simulink model "Problema4"  (R2023b)
settings: Solver=ode45  StartTime=0  StopTime=50  FixedStep=1  RelTol=1e-3
values from neighbouring files (symbols this model uses):
  constants = {    [sim_utils.m]
settings Model: Creator=alfre  LastModifiedBy=alfre

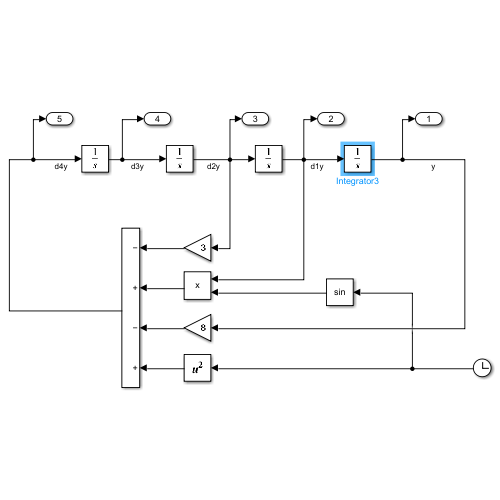
[thumbnail: Simulink's stored preview of the top-level diagram]
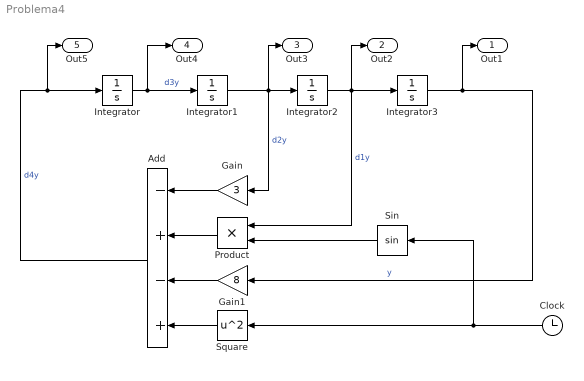
== system Problema4 ==
  Add : Sum  Inputs=-+-+
  Clock : Clock
  Gain : Gain  Gain=3
  Gain1 : Gain  Gain=8
  Integrator : Integrator  InitialCondition=constants{1}.d3y0
  Integrator1 : Integrator  InitialCondition=constants{1}.d2y0
  Integrator2 : Integrator  InitialCondition=constants{1}.dy0
  Integrator3 : Integrator  InitialCondition=constants{1}.y0
  Product : Product
  Sin : Trigonometry
  Square : Math  Operator=square
  Out1 : Outport
  Out2 : Outport  Port=2
  Out3 : Outport  Port=3
  Out4 : Outport  Port=4
  Out5 : Outport  Port=5
  wires:
  Integrator/1 -> Out4/1, Integrator1/1  "d3y"
  Integrator1/1 -> Out3/1, Gain/1, Integrator2/1  "d2y"
  Integrator2/1 -> Out2/1, Product/1, Integrator3/1  "d1y"
  Integrator3/1 -> Out1/1, Gain1/1  "y"
  Add/1 -> Out5/1, Integrator/1  "d4y"
  Gain/1 -> Add/1
  Clock/1 -> Square/1, Sin/1
  Sin/1 -> Product/2
  Product/1 -> Add/2
  Gain1/1 -> Add/3
  Square/1 -> Add/4
